simulink model "Hill_muscle_model_simulink"  (R2019a)
settings: Solver=ode45  StartTime=0.0  StopTime=2  FixedStep=0.0001  MaxStep=0.1  RelTol=1e-6  EnableMultiTasking=on
undefined symbols (not defined in the file): prop
(part 1 of 3)
settings Model: Creator=uqglicht  LastModifiedBy=deanm
settings DataIOCC: SaveFormat=Array  SignalLoggingSaveFormat=ModelDataLogs  ReturnWorkspaceOutputs=off
settings OptimizationCC: ExpressionDepthLimit=2147483647  LifeSpan=inf
settings DebuggingCC: AlgebraicLoopMsg=none  UnderspecifiedInitializationDetection=Classic  MergeDetectMultiDrivingBlocksExec=none  FcnCallInpInsideContextMsg=warning  StateNameClashWarn=warning  SFUnexpectedBacktrackingDiag=warning  SFNoUnconditionalDefaultTransitionDiag=warning  SFExecutionAtInitializationDiag=none  ArithmeticOperatorsInVariantConditions=warning
settings HardwareCC: ProdBitPerPointer=32  ProdBitPerSizeT=32  ProdBitPerPtrDiffT=32  ProdLargestAtomicFloat=None  ProdIntDivRoundTo=Undefined  ProdEndianess=Unspecified  ProdWordSize=32  ProdHWDeviceType=32-bit Generic
settings ModelReferenceCC: PropagateSignalLabelsOutOfModel=off
settings SFSimCC: SimUseLocalCustomCode=off
settings RTWCC: RTWUseLocalCustomCode=off
settings CodeAppCC: StateflowObjectComments=on
settings GRTTargetCC: TargetLangStandard=C89/C90 (ANSI)  CombineOutputUpdateFcns=off  GRTInterface=on
settings ConfigComp: CovMetricSettings=dw  CovSaveCumulativeToWorkspaceVar=on  CovSaveSingleToWorkspaceVar=on  CovExternalEMLEnable=off

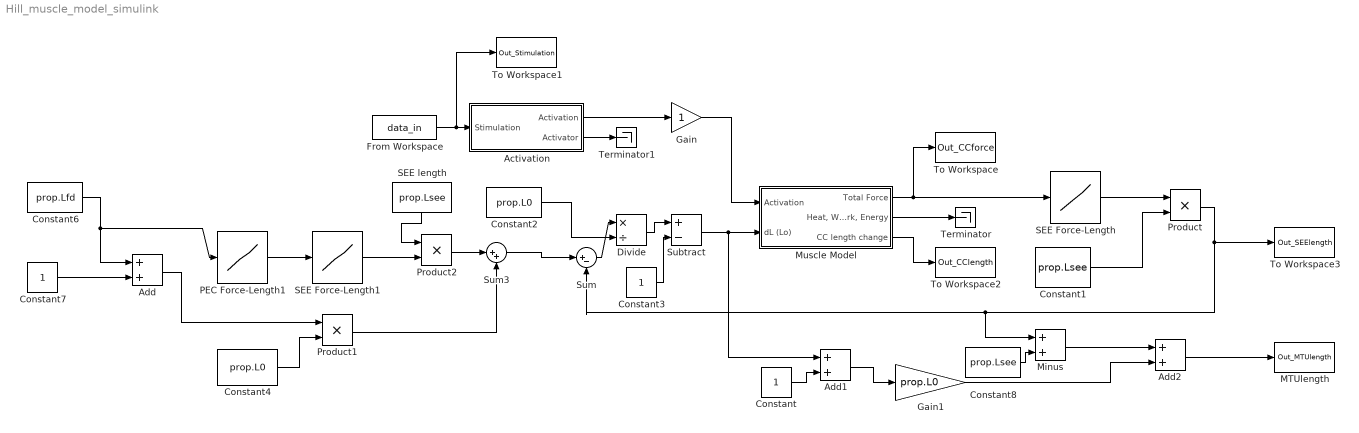
== system Hill_muscle_model_simulink ==
  " PEC Force-Length1" : Lookup  InputValues=|  Table=|  LookUpMeth=Interpolation-Use End Values  SaturateOnIntegerOverflow=on
      InputValues=|
      | [-0.400000000000000
      | -0.200000000000000
      | -0.0200000000000000
      | -0.0181000000000000
      | -0.0162000000000000
      | -0.0143000000000000
      | -0.0124000000000000
      | -0.0105000000000001
      | -0.00860000000000005
      | -0.00670000000000004
      | -0.00480000000000003
      | -0.00290000000000001
      | -0.00100000000000000
      | 0.000899999999999901
      | 0.00279999999999991
      | 0.00469999999999993
      | 0.00659999999999994
      | 0.00849999999999995
      | 0.0104000000000000
      | 0.0123000000000000
      | 0.0142000000000000
      | 0.0161000000000000
      | 0.0180000000000000
      | 0.0199000000000000
      | 0.0218000000000000
      | 0.0237000000000001
      | 0.0256000000000001
      | 0.0274999999999999
      | 0.0293999999999999
      | 0.0312999999999999
      | 0.0331999999999999
      | 0.0350999999999999
      | 0.0369999999999999
      | 0.0388999999999999
      | 0.0408000000000000
      | 0.0427000000000000
      | 0.0446000000000000
      | 0.0465000000000000
      | 0.0484000000000000
      | 0.0503000000000000
      | 0.0522000000000000
      | 0.0541000000000000
      | 0.0560000000000001
      | 0.0579000000000001
      | 0.0598000000000001
      | 0.0616999999999999
      | 0.0635999999999999
      | 0.0654999999999999
      | 0.0673999999999999
      | 0.0692999999999999
      | 0.0711999999999999
      | 0.0730999999999999
      | 0.0750000000000000
      | 0.0769000000000000
      | 0.0788000000000000
      | 0.0807000000000000
      | 0.0826000000000000
      | 0.0845000000000000
      | 0.0864000000000000
      | 0.0883000000000001
      | 0.0901999999999998
      | 0.0920999999999999
      | 0.0939999999999999
      | 0.0958999999999999
      | 0.0977999999999999
      | 0.0996999999999999
      | 0.101600000000000
      | 0.103500000000000
      | 0.105400000000000
      | 0.107300000000000
      | 0.109200000000000
      | 0.111100000000000
      | 0.113000000000000
      | 0.114900000000000
      | 0.116800000000000
      | 0.118700000000000
      | 0.120600000000000
      | 0.122500000000000
      | 0.124400000000000
      | 0.126300000000000
      | 0.128200000000000
      | 0.130100000000000
      | 0.132000000000000
      | 0.133900000000000
      | 0.135800000000000
      | 0.137700000000000
      | 0.139600000000000
      | 0.141500000000000
      | 0.143400000000000
      | 0.145300000000000
      | 0.147200000000000
      | 0.149100000000000
      | 0.151000000000000
      | 0.152900000000000
      | 0.154800000000000
      | 0.156700000000000
      | 0.158600000000000
      | 0.160500000000000
      | 0.162400000000000
      | 0.164300000000000
      | 0.166200000000000
      | 0.168100000000000
      | 0.170000000000000
      | 0.171900000000000
      | 0.173800000000000
      | 0.175700000000000
      | 0.177600000000000
      | 0.179500000000000
      | 0.181400000000000
      | 0.183300000000000
      | 0.185200000000000
      | 0.187100000000000
      | 0.189000000000000
      | 0.190900000000000
      | 0.192800000000000
      | 0.194700000000000
      | 0.196600000000000
      | 0.198500000000000
      | 0.200400000000000
      | 0.202300000000000
      | 0.204200000000000
      | 0.206100000000000
      | 0.208000000000000
      | 0.209900000000000
      | 0.211800000000000
      | 0.213700000000000
      | 0.215600000000000
      | 0.217500000000000
      | 0.219400000000000
      | 0.221300000000000
      | 0.223200000000000
      | 0.225100000000000
      | 0.227000000000000
      | 0.228900000000000
      | 0.230800000000000
      | 0.232700000000000
      | 0.234600000000000
      | 0.236500000000000
      | 0.238400000000000
      | 0.240300000000000
      | 0.242200000000000
      | 0.244100000000000
      | 0.246000000000000
      | 0.247900000000000
      | 0.249800000000000
      | 0.251700000000000
      | 0.253600000000000
      | 0.255500000000000
      | 0.257400000000000
      | 0.259300000000000
      | 0.261200000000000
      | 0.263100000000000
      | 0.265000000000000
      | 0.266900000000000
      | 0.268800000000000
      | 0.270700000000000
      | 0.272600000000000
      | 0.274500000000000
      | 0.276400000000000
      | 0.278300000000000
      | 0.280200000000000
      | 0.282100000000000
      | 0.284000000000000
      | 0.285900000000000
      | 0.287800000000000
      | 0.289700000000000
      | 0.291600000000000
      | 0.293500000000000
      | 0.295400000000000
      | 0.297300000000000
      | 0.299200000000000
      | 0.301100000000000
      | 0.303000000000000
      | 0.304900000000000
      | 0.306800000000000
      | 0.308700000000000
      | 0.310600000000000
      | 0.312500000000000
      | 0.314400000000000
      | 0.316300000000000
      | 0.318200000000000
      | 0.320100000000000
      | 0.322000000000000
      | 0.323900000000000
      | 0.325800000000000
      | 0.327700000000000
      | 0.329600000000000
      | 0.331500000000000
      | 0.333400000000000
      | 0.335300000000000
      | 0.337200000000000
      | 0.339100000000000
      | 0.341000000000000
      | 0.342900000000000
      | 0.344800000000000
      | 0.346700000000000
      | 0.348600000000000
      | 0.350500000000000
      | 0.352400000000000
      | 0.354300000000000
      | 0.356200000000000
      | 0.358100000000000
      | 0.360000000000000
      | 0.361900000000000
      | 0.363800000000000
      | 0.365700000000000
      | 0.367600000000000
      | 0.369500000000000
      | 0.371400000000000
      | 0.373300000000000
      | 0.375200000000000
      | 0.377100000000000
      | 0.379000000000000
      | 0.380900000000000
      | 0.382800000000000
      | 0.384700000000000
      | 0.386600000000000
      | 0.388500000000000
      | 0.390400000000000
      | 0.392300000000000
      | 0.394200000000000
      | 0.396100000000000
      | 0.398000000000000
      | 0.399900000000000
      | 0.401800000000000
      | 0.403700000000000
      | 0.405600000000000
      | 0.407500000000000
      | 0.409400000000000
      | 0.411300000000000
      | 0.413200000000000
      | 0.415100000000000
      | 0.417000000000000
      | 0.418900000000000
      | 0.420800000000000
      | 0.422700000000000
      | 0.424600000000000
      | 0.426500000000000
      | 0.428400000000000
      | 0.430300000000000
      | 0.432200000000000
      | 0.434100000000000
      | 0.436000000000000
      | 0.437900000000000
      | 0.439800000000000
      | 0.441700000000000
      | 0.443600000000000
      | 0.445500000000000
      | 0.447400000000000
      | 0.449300000000000
      | 0.451200000000000
      | 0.453100000000000
      | 0.455000000000000
      | 0.456900000000000
      | 0.458800000000000
      | 0.460700000000000
      | 0.462600000000000
      | 0.464500000000000
      | 0.466400000000000
      | 0.468300000000000
      | 0.470200000000000
      | 0.472100000000000
      | 0.474000000000000
      | 0.475900000000000
      | 0.477800000000000
      | 0.479700000000000
      | 0.481600000000000
      | 0.483500000000000
      | 0.485400000000000
      | 0.487300000000000
      | 0.489200000000000
      | 0.491100000000000
      | 0.493000000000000
      | 0.494900000000000
      | 0.496800000000000
      | 0.498700000000000
      | 0.500600000000000
      | 0.502500000000000
      | 0.504400000000000
      | 0.506300000000000
      | 0.508200000000000
      | 0.510100000000000
      | 0.512000000000000
      | 0.513900000000000
      | 0.515800000000000
      | 0.517700000000000
      | 0.519600000000000
      | 0.521500000000000
      | 0.523400000000000
      | 0.525300000000000
      | 0.527200000000000
      | 0.529100000000000
      | 0.531000000000000
      | 0.532900000000000
      | 0.534800000000000
      | 0.536700000000000
      | 0.538600000000000
      | 0.540500000000000
      | 0.542400000000000
      | 0.544300000000000
      | 0.546200000000000
      | 0.548100000000000
      | 0.550000000000000]
      Table=|
      | [0
      | 0
      | 0
      | 0.000250430632326719
      | 0.000504222699518002
      | 0.000761421320832001
      | 0.00102207222114546
      | 0.00128622173908269
      | 0.00155391683525374
      | 0.00182520510060293
      | 0.00210013476486974
      | 0.00237875470516303
      | 0.00266111445465043
      | 0.00294726421136441
      | 0.00323725484712650
      | 0.00353113791659126
      | 0.00382896566641171
      | 0.00413079104452780
      | 0.00443666770957945
      | 0.00474665004044605
      | 0.00506079314591397
      | 0.00537915287447376
      | 0.00570178582424899
      | 0.00602874935305825
      | 0.00636010158861225
      | 0.00669590143884778
      | 0.00703620860240042
      | 0.00738108357921772
      | 0.00773058768131505
      | 0.00808478304367549
      | 0.00844373263529632
      | 0.00880750027038366
      | 0.00917615061969739
      | 0.00954974922204830
      | 0.00992836249594969
      | 0.0103120577514252
      | 0.0107009032019753
      | 0.0110949679767041
      | 0.0114943221326095
      | 0.0118990366670377
      | 0.0123091835303051
      | 0.0127248356384900
      | 0.0131460668863951
      | 0.0135729521606851
      | 0.0140055673531997
      | 0.0144439893744458
      | 0.0148882961672708
      | 0.0153385667207193
      | 0.0157948810840755
      | 0.0162573203810947
      | 0.0167259668244255
      | 0.0172009037302254
      | 0.0176822155329729
      | 0.0181699878004785
      | 0.0186643072490966
      | 0.0191652617591422
      | 0.0196729403905143
      | 0.0201874333985288
      | 0.0207088322499646
      | 0.0212372296393239
      | 0.0217727195053120
      | 0.0223153970475379
      | 0.0228653587434382
      | 0.0234227023654295
      | 0.0239875269982905
      | 0.0245599330567766
      | 0.0251400223034726
      | 0.0257278978668835
      | 0.0263236642597689
      | 0.0269274273977232
      | 0.0275392946180057
      | 0.0281593746986226
      | 0.0287877778776657
      | 0.0294246158729108
      | 0.0300700019016789
      | 0.0307240507009637
      | 0.0313868785478300
      | 0.0320586032800850
      | 0.0327393443172282
      | 0.0334292226816813
      | 0.0341283610203039
      | 0.0348368836261974
      | 0.0355549164608025
      | 0.0362825871762918
      | 0.0370200251382647
      | 0.0377673614487455
      | 0.0385247289694911
      | 0.0392922623456110
      | 0.0400700980295046
      | 0.0408583743051200
      | 0.0416572313125378
      | 0.0424668110728856
      | 0.0432872575135862
      | 0.0441187164939458
      | 0.0449613358310838
      | 0.0458152653262129
      | 0.0466806567912702
      | 0.0475576640759063
      | 0.0484464430948374
      | 0.0493471518555631
      | 0.0502599504864576
      | 0.0511850012652372
      | 0.0521224686478100
      | 0.0530725192975131
      | 0.0540353221147419
      | 0.0550110482669776
      | 0.0559998712192171
      | 0.0570019667648116
      | 0.0580175130567198
      | 0.0590466906391794
      | 0.0600896824798044
      | 0.0611466740021136
      | 0.0622178531184946
      | 0.0633034102636119
      | 0.0644035384282613
      | 0.0655184331936807
      | 0.0666482927663203
      | 0.0677933180130799
      | 0.0689537124970191
      | 0.0701296825135468
      | 0.0713214371270965
      | 0.0725291882082938
      | 0.0737531504716231
      | 0.0749935415135991
      | 0.0762505818514518
      | 0.0775244949623297
      | 0.0788155073230299
      | 0.0801238484502616
      | 0.0814497509414482
      | 0.0827934505160806
      | 0.0841551860576222
      | 0.0855351996559779
      | 0.0869337366505331
      | 0.0883510456737703
      | 0.0897873786954709
      | 0.0912429910675106
      | 0.0927181415692559
      | 0.0942130924535702
      | 0.0957281094934369
      | 0.0972634620292087
      | 0.0988194230164915
      | 0.100396269074670
      | 0.101994280536085
      | 0.103613741495872
      | 0.105254939862466
      | 0.106918167408790
      | 0.108603719824120
      | 0.110311896766659
      | 0.112043001916806
      | 0.113797343031148
      | 0.115575231997169
      | 0.117376984888702
      | 0.119202922022118
      | 0.121053368013270
      | 0.122928651835210
      | 0.124829106876667
      | 0.126755071001320
      | 0.128706886607864
      | 0.130684900690880
      | 0.132689464902527
      | 0.134720935615054
      | 0.136779673984162
      | 0.138866046013205
      | 0.140980422618260
      | 0.143123179694070
      | 0.145294698180871
      | 0.147495364132113
      | 0.149725568783094
      | 0.151985708620514
      | 0.154276185452965
      | 0.156597406482360
      | 0.158949784376328
      | 0.161333737341581
      | 0.163749689198257
      | 0.166198069455271
      | 0.168679313386674
      | 0.171193862109033
      | 0.173742162659853
      | 0.176324668077057
      | 0.178941837479519
      | 0.181594136148693
      | 0.184282035611329
      | 0.187006013723299
      | 0.189766554754552
      | 0.192564149475209
      | 0.195399295242811
      | 0.198272496090739
      | 0.201184262817823
      | 0.204135113079149
      | 0.207125571478092
      | 0.210156169659575
      | 0.213227446404592
      | 0.216339947725985
      | 0.219494226965522
      | 0.222690844892261
      | 0.225930369802255
      | 0.229213377619576
      | 0.232540451998703
      | 0.235912184428290
      | 0.239329174336315
      | 0.242792029196650
      | 0.246301364637058
      | 0.249857804548637
      | 0.253461981196739
      | 0.257114535333370
      | 0.260816116311110
      | 0.264567382198546
      | 0.268368999897273
      | 0.272221645260450
      | 0.276126003212955
      | 0.280082767873150
      | 0.284092642676287
      | 0.288156340499557
      | 0.292274583788832
      | 0.296448104687099
      | 0.300677645164621
      | 0.304963957150844
      | 0.309307802668078
      | 0.313709953966966
      | 0.318171193663777
      | 0.322692314879541
      | 0.327274121381048
      | 0.331917427723744
      | 0.336623059396541
      | 0.341391852968574
      | 0.346224656237928
      | 0.351122328382355
      | 0.356085740112027
      | 0.361115773824323
      | 0.366213323760705
      | 0.371379296165701
      | 0.376614609448009
      | 0.381920194343780
      | 0.387296994082079
      | 0.392745964552578
      | 0.398268074475489
      | 0.403864305573786
      | 0.409535652747737
      | 0.415283124251777
      | 0.421107741873755
      | 0.427010541116590
      | 0.432992571382358
      | 0.439054896158864
      | 0.445198593208700
      | 0.451424754760857
      | 0.457734487704898
      | 0.464128913787741
      | 0.470609169813088
      | 0.477176407843523
      | 0.483831795405323
      | 0.490576515696030
      | 0.497411767794791
      | 0.504338766875539
      | 0.511358744423021
      | 0.518472948451733
      | 0.525682643727797
      | 0.532989111993804
      | 0.540393652196691
      | 0.547897580718662
      | 0.555502231611216
      | 0.563208956832321
      | 0.571019126486758
      | 0.578934129069701
      | 0.586955371713568
      | 0.595084280438176
      | 0.603322300404264
      | 0.611670896170412
      | 0.620131551953410
      | 0.628705771892127
      | 0.637395080314910
      | 0.646201022010589
      | 0.655125162503100
      | 0.664169088329814
      | 0.673334407323585
      | 0.682622748898598
      | 0.692035764340038
      | 0.701575127097666
      | 0.711242533083318
      | 0.721039700972408
      | 0.730968372509477
      | 0.741030312817836
      | 0.751227310713372
      | 0.761561179022571
      | 0.772033754904790
      | 0.782646900178882
      | 0.793402501654181
      | 0.804302471465943
      | 0.815348747415287
      | 0.826543293313698
      | 0.837888099332151
      | 0.849385182354932
      | 0.861036586338189
      | 0.872844382673316
      | 0.884810670555210
      | 0.896937577355452
      | 0.909227259000524
      | 0.921681900355087
      | 0.934303715610405
      | 0.947094948677991
      | 0.960057873588522
      | 0.973194794896123
      | 0.986508048088072
      | 0.999999999999999]
  " SEE Force-Length" : Lookup  InputValues=|  Table=|  SaturateOnIntegerOverflow=on
      InputValues=|
      | [0
      | 0.000442588372362627
      | 0.00141523090125158
      | 0.00279339495313245
      | 0.00452537533502198
      | 0.00657919407104800
      | 0.00893222484804500
      | 0.0115672311194430
      | 0.0144704457093994
      | 0.0176305024068561
      | 0.0210377843976648
      | 0.0246839997310470
      | 0.0285618904861856
      | 0.0326650255195540
      | 0.0369876479916691
      | 0.0415245602039597
      | 0.0462710346715712
      | 0.0512227441486924
      | 0.0563757056643364
      | 0.0617262351241129
      | 0.0672709100207659
      | 0.0730065384643556
      | 0.0789301332056712
      | 0.0850388896535411
      | 0.0913301671221823
      | 0.0978014727170639
      | 0.104450447395775
      | 0.111274853836761
      | 0.118272565822261
      | 0.125441558898393
      | 0.132779902119470
      | 0.140285750718276
      | 0.147957339571581
      | 0.155792977352181
      | 0.163791041276471
      | 0.171949972371004
      | 0.180268271193222
      | 0.188744493951255
      | 0.197377248975694
      | 0.206165193502878
      | 0.215107030734867
      | 0.224201507145885
      | 0.233447410009032
      | 0.242843565120379
      | 0.252388834700443
      | 0.262082115455459
      | 0.271922336782965
      | 0.281908459108055
      | 0.292039472338153
      | 0.302314394425579
      | 0.312732270028317
      | 0.323292169260420
      | 0.333993186524427
      | 0.344834439418896
      | 0.355815067714905
      | 0.366934232395953
      | 0.378191114756247
      | 0.389584915552842
      | 0.401114854207514
      | 0.412780168054648
      | 0.424580111631741
      | 0.436513956009434
      | 0.448580988158254
      | 0.460780510349489
      | 0.473111839587851
      | 0.485574307073750
      | 0.498167257693216
      | 0.510890049533639
      | 0.523742053423653
      | 0.536722652495622
      | 0.549831241769308
      | 0.563067227755399
      | 0.576430028077688
      | 0.589919071112773
      | 0.603533795646242
      | 0.617273650544365
      | 0.631138094440404
      | 0.645126595434705
      | 0.659238630807786
      | 0.673473686745707
      | 0.687831258077046
      | 0.702310848020841
      | 0.716911967944929
      | 0.731634137134105
      | 0.746476882567616
      | 0.761439738705489
      | 0.776522247283244
      | 0.791723957114576
      | 0.807044423901603
      | 0.822483210052306
      | 0.838039884504814
      | 0.853714022558200
      | 0.869505205709484
      | 0.885413021496541
      | 0.901437063346643
      | 0.917576930430383
      | 0.933832227520716
      | 0.950202564856904
      | 0.966687558013140
      | 0.983286827771638
      | 1]
      Table=|
      | [0
      | 0.000500000000000000
      | 0.00100000000000000
      | 0.00150000000000000
      | 0.00200000000000000
      | 0.00250000000000000
      | 0.00300000000000000
      | 0.00350000000000000
      | 0.00400000000000000
      | 0.00450000000000000
      | 0.00500000000000000
      | 0.00550000000000000
      | 0.00600000000000000
      | 0.00650000000000000
      | 0.00700000000000000
      | 0.00750000000000000
      | 0.00800000000000000
      | 0.00850000000000000
      | 0.00900000000000000
      | 0.00950000000000000
      | 0.0100000000000000
      | 0.0105000000000000
      | 0.0110000000000000
      | 0.0115000000000000
      | 0.0120000000000000
      | 0.0125000000000000
      | 0.0130000000000000
      | 0.0135000000000000
      | 0.0140000000000000
      | 0.0145000000000000
      | 0.0150000000000000
      | 0.0155000000000000
      | 0.0160000000000000
      | 0.0165000000000000
      | 0.0170000000000000
      | 0.0175000000000000
      | 0.0180000000000000
      | 0.0185000000000000
      | 0.0190000000000000
      | 0.0195000000000000
      | 0.0200000000000000
      | 0.0205000000000000
      | 0.0210000000000000
      | 0.0215000000000000
      | 0.0220000000000000
      | 0.0225000000000000
      | 0.0230000000000000
      | 0.0235000000000000
      | 0.0240000000000000
      | 0.0245000000000000
      | 0.0250000000000000
      | 0.0255000000000000
      | 0.0260000000000000
      | 0.0265000000000000
      | 0.0270000000000000
      | 0.0275000000000000
      | 0.0280000000000000
      | 0.0285000000000000
      | 0.0290000000000000
      | 0.0295000000000000
      | 0.0300000000000000
      | 0.0305000000000000
      | 0.0310000000000000
      | 0.0315000000000000
      | 0.0320000000000000
      | 0.0325000000000000
      | 0.0330000000000000
      | 0.0335000000000000
      | 0.0340000000000000
      | 0.0345000000000000
      | 0.0350000000000000
      | 0.0355000000000000
      | 0.0360000000000000
      | 0.0365000000000000
      | 0.0370000000000000
      | 0.0375000000000000
      | 0.0380000000000000
      | 0.0385000000000000
      | 0.0390000000000000
      | 0.0395000000000000
      | 0.0400000000000000
      | 0.0405000000000000
      | 0.0410000000000000
      | 0.0415000000000000
      | 0.0420000000000000
      | 0.0425000000000000
      | 0.0430000000000000
      | 0.0435000000000000
      | 0.0440000000000000
      | 0.0445000000000000
      | 0.0450000000000000
      | 0.0455000000000000
      | 0.0460000000000000
      | 0.0465000000000000
      | 0.0470000000000000
      | 0.0475000000000000
      | 0.0480000000000000
      | 0.0485000000000000
      | 0.0490000000000000
      | 0.0495000000000000
      | 0.0500000000000000]*prop.NewTL
  Activation : Subsystem
  Add : Sum
  Add1 : Sum
  Add2 : Sum
  Constant : Constant
  Constant1 : Constant  Value=prop.Lsee
  Constant2 : Constant  Value=prop.L0
  Constant3 : Constant
  Constant4 : Constant  Value=prop.L0
  Constant6 : Constant  Value=prop.Lfd
  Constant7 : Constant
  Constant8 : Constant  Value=prop.Lsee
  Divide : Product  Inputs=*/
  From Workspace : FromWorkspace  VariableName=data_in  SampleTime=1/10000
  Gain : Gain
  Gain1 : Gain  Gain=prop.L0
  MTUlength : ToWorkspace  VariableName=Out_MTUlength  SaveFormat=Structure With Time  SampleTime=-1
  Minus : Sum
  Muscle Model : Subsystem
  Product : Product
  Product1 : Product
  Product2 : Product
  SEE Force-Length1 : Lookup  InputValues=|  Table=|  SaturateOnIntegerOverflow=on
      InputValues=|
      | [0
      | 0.000442588372362627
      | 0.00141523090125158
      | 0.00279339495313245
      | 0.00452537533502198
      | 0.00657919407104800
      | 0.00893222484804500
      | 0.0115672311194430
      | 0.0144704457093994
      | 0.0176305024068561
      | 0.0210377843976648
      | 0.0246839997310470
      | 0.0285618904861856
      | 0.0326650255195540
      | 0.0369876479916691
      | 0.0415245602039597
      | 0.0462710346715712
      | 0.0512227441486924
      | 0.0563757056643364
      | 0.0617262351241129
      | 0.0672709100207659
      | 0.0730065384643556
      | 0.0789301332056712
      | 0.0850388896535411
      | 0.0913301671221823
      | 0.0978014727170639
      | 0.104450447395775
      | 0.111274853836761
      | 0.118272565822261
      | 0.125441558898393
      | 0.132779902119470
      | 0.140285750718276
      | 0.147957339571581
      | 0.155792977352181
      | 0.163791041276471
      | 0.171949972371004
      | 0.180268271193222
      | 0.188744493951255
      | 0.197377248975694
      | 0.206165193502878
      | 0.215107030734867
      | 0.224201507145885
      | 0.233447410009032
      | 0.242843565120379
      | 0.252388834700443
      | 0.262082115455459
      | 0.271922336782965
      | 0.281908459108055
      | 0.292039472338153
      | 0.302314394425579
      | 0.312732270028317
      | 0.323292169260420
      | 0.333993186524427
      | 0.344834439418896
      | 0.355815067714905
      | 0.366934232395953
      | 0.378191114756247
      | 0.389584915552842
      | 0.401114854207514
      | 0.412780168054648
      | 0.424580111631741
      | 0.436513956009434
      | 0.448580988158254
      | 0.460780510349489
      | 0.473111839587851
      | 0.485574307073750
      | 0.498167257693216
      | 0.510890049533639
      | 0.523742053423653
      | 0.536722652495622
      | 0.549831241769308
      | 0.563067227755399
      | 0.576430028077688
      | 0.589919071112773
      | 0.603533795646242
      | 0.617273650544365
      | 0.631138094440404
      | 0.645126595434705
      | 0.659238630807786
      | 0.673473686745707
      | 0.687831258077046
      | 0.702310848020841
      | 0.716911967944929
      | 0.731634137134105
      | 0.746476882567616
      | 0.761439738705489
      | 0.776522247283244
      | 0.791723957114576
      | 0.807044423901603
      | 0.822483210052306
      | 0.838039884504814
      | 0.853714022558200
      | 0.869505205709484
      | 0.885413021496541
      | 0.901437063346643
      | 0.917576930430383
      | 0.933832227520716
      | 0.950202564856904
      | 0.966687558013140
      | 0.983286827771638
      | 1]
      Table=|
      | [0
      | 0.000500000000000000
      | 0.00100000000000000
      | 0.00150000000000000
      | 0.00200000000000000
      | 0.00250000000000000
      | 0.00300000000000000
      | 0.00350000000000000
      | 0.00400000000000000
      | 0.00450000000000000
      | 0.00500000000000000
      | 0.00550000000000000
      | 0.00600000000000000
      | 0.00650000000000000
      | 0.00700000000000000
      | 0.00750000000000000
      | 0.00800000000000000
      | 0.00850000000000000
      | 0.00900000000000000
      | 0.00950000000000000
      | 0.0100000000000000
      | 0.0105000000000000
      | 0.0110000000000000
      | 0.0115000000000000
      | 0.0120000000000000
      | 0.0125000000000000
      | 0.0130000000000000
      | 0.0135000000000000
      | 0.0140000000000000
      | 0.0145000000000000
      | 0.0150000000000000
      | 0.0155000000000000
      | 0.0160000000000000
      | 0.0165000000000000
      | 0.0170000000000000
      | 0.0175000000000000
      | 0.0180000000000000
      | 0.0185000000000000
      | 0.0190000000000000
      | 0.0195000000000000
      | 0.0200000000000000
      | 0.0205000000000000
      | 0.0210000000000000
      | 0.0215000000000000
      | 0.0220000000000000
      | 0.0225000000000000
      | 0.0230000000000000
      | 0.0235000000000000
      | 0.0240000000000000
      | 0.0245000000000000
      | 0.0250000000000000
      | 0.0255000000000000
      | 0.0260000000000000
      | 0.0265000000000000
      | 0.0270000000000000
      | 0.0275000000000000
      | 0.0280000000000000
      | 0.0285000000000000
      | 0.0290000000000000
      | 0.0295000000000000
      | 0.0300000000000000
      | 0.0305000000000000
      | 0.0310000000000000
      | 0.0315000000000000
      | 0.0320000000000000
      | 0.0325000000000000
      | 0.0330000000000000
      | 0.0335000000000000
      | 0.0340000000000000
      | 0.0345000000000000
      | 0.0350000000000000
      | 0.0355000000000000
      | 0.0360000000000000
      | 0.0365000000000000
      | 0.0370000000000000
      | 0.0375000000000000
      | 0.0380000000000000
      | 0.0385000000000000
      | 0.0390000000000000
      | 0.0395000000000000
      | 0.0400000000000000
      | 0.0405000000000000
      | 0.0410000000000000
      | 0.0415000000000000
      | 0.0420000000000000
      | 0.0425000000000000
      | 0.0430000000000000
      | 0.0435000000000000
      | 0.0440000000000000
      | 0.0445000000000000
      | 0.0450000000000000
      | 0.0455000000000000
      | 0.0460000000000000
      | 0.0465000000000000
      | 0.0470000000000000
      | 0.0475000000000000
      | 0.0480000000000000
      | 0.0485000000000000
      | 0.0490000000000000
      | 0.0495000000000000
      | 0.0500000000000000]*prop.NewTL
  SEE length : Constant  Value=prop.Lsee
  Subtract : Sum  Inputs=+-
  Sum : Sum  Inputs=|+-
  Sum3 : Sum  Inputs=|++
  Terminator : Terminator
  Terminator1 : Terminator
  To Workspace : ToWorkspace  VariableName=Out_CCforce  SaveFormat=Structure  SampleTime=-1
  To Workspace1 : ToWorkspace  VariableName=Out_Stimulation  SaveFormat=Structure  SampleTime=-1
  To Workspace2 : ToWorkspace  VariableName=Out_CClength  SaveFormat=Structure With Time  SampleTime=-1
  To Workspace3 : ToWorkspace  VariableName=Out_SEElength  SaveFormat=Structure With Time  SampleTime=-1
  wires:
  Muscle Model/1(Total Force) -> " SEE Force-Length"/1, To Workspace/1
  Activation/1(Activation) -> Gain/1
  From Workspace/1 -> To Workspace1/1, Activation/1(Stimulation)
  Muscle Model/3(CC length change) -> To Workspace2/1
  Muscle Model/2("Heat, Work, Energy") -> Terminator/1
  " SEE Force-Length"/1 -> Product/1
  Constant1/1 -> Product/2
  Constant2/1 -> Divide/2
  Sum/1 -> Divide/1
  Divide/1 -> Subtract/1
  Constant3/1 -> Subtract/2
  " PEC Force-Length1"/1 -> SEE Force-Length1/1
  Constant4/1 -> Product1/2
  SEE length/1 -> Product2/1
  Product2/1 -> Sum3/1
  Product1/1 -> Sum3/2
  Constant6/1 -> Add/1, " PEC Force-Length1"/1
  Constant7/1 -> Add/2
  Add/1 -> Product1/1
  Sum3/1 -> Sum/1
  Product/1 -> Minus/1, Sum/2, To Workspace3/1
  Gain/1 -> Muscle Model/1(Activation)
  Subtract/1 -> Add1/1, Muscle Model/2(dL (Lo))
  Constant/1 -> Add1/2
  Constant8/1 -> Minus/2
  Minus/1 -> Add2/1
  Add2/1 -> MTUlength/1
  Add1/1 -> Gain1/1
  Gain1/1 -> Add2/2
  SEE Force-Length1/1 -> Product2/2
  Activation/2(Activator) -> Terminator1/1

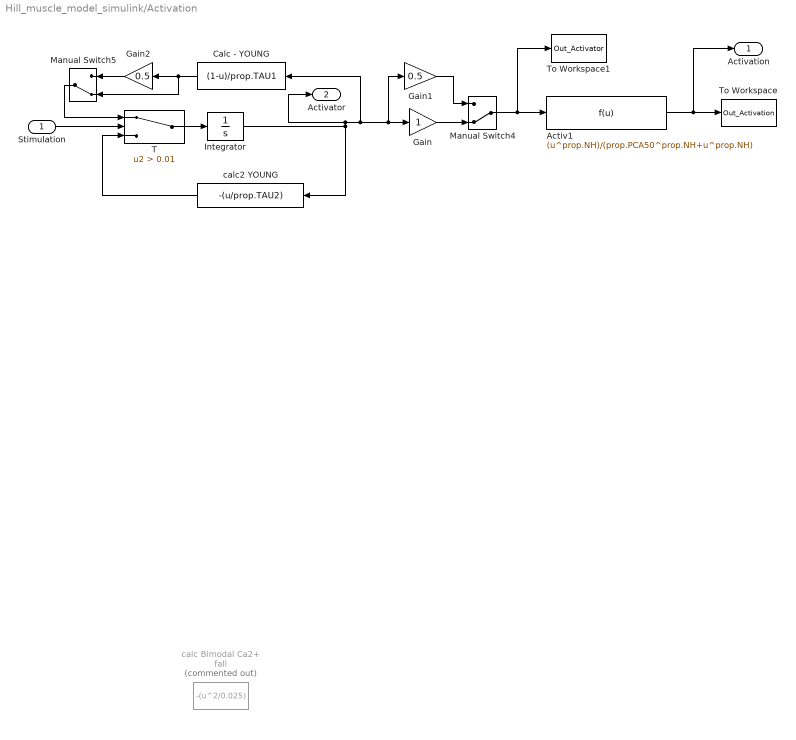
== system Hill_muscle_model_simulink/Activation ==
  Stimulation : Inport
  Activ1 : Fcn  Expr=(u^prop.NH)/(prop.PCA50^prop.NH+u^prop.NH)
  Calc - YOUNG : Fcn  Expr=(1-u)/prop.TAU1
  Gain : Gain
  Gain1 : Gain  Gain=0.5
  Gain2 : Gain  Gain=0.5
  Integrator : Integrator
  Manual Switch4 : ManualSwitch  CurrentSetting=0
  Manual Switch5 : ManualSwitch  CurrentSetting=0
  T : Switch  Criteria=u2 > Threshold  Threshold=0.01  SaturateOnIntegerOverflow=on  InputSameDT=on
  To Workspace : ToWorkspace  VariableName=Out_Activation  SaveFormat=Structure  SampleTime=-1
  To Workspace1 : ToWorkspace  VariableName=Out_Activator  SaveFormat=Structure  SampleTime=-1
  calc Bimodal Ca2+ fall : Fcn  Commented=on  Expr=-(u^2/0.025)
  calc2 YOUNG : Fcn  Expr=-(u/prop.TAU2)
  Activation : Outport
  Activator : Outport  Port=2
  wires:
  T/1 -> Integrator/1
  Stimulation/1 -> T/2
  Calc - YOUNG/1 -> Manual Switch5/2, Gain2/1
  calc2 YOUNG/1 -> T/3
  Integrator/1 -> calc2 YOUNG/1, Gain1/1, Gain/1, Calc - YOUNG/1, Activator/1
  Gain/1 -> Manual Switch4/2
  Gain1/1 -> Manual Switch4/1
  Gain2/1 -> Manual Switch5/1
  Manual Switch5/1 -> T/1
  Manual Switch4/1 -> To Workspace1/1, Activ1/1
  Activ1/1 -> Activation/1, To Workspace/1
